simulink model "linearSingleTrack_SchrammHiller"  (R2018b)
settings: Solver=VariableStepAuto  StartTime=0.0  StopTime=20  RelTol=1e-3
settings Model: Creator=utente  LastModifiedBy=utente

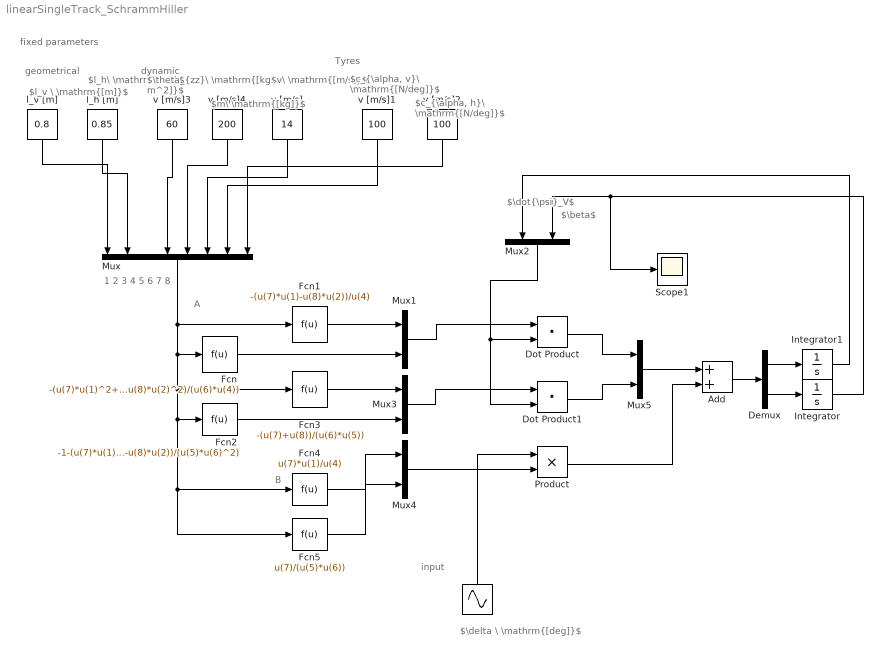
== system linearSingleTrack_SchrammHiller ==
  note: A
  note: B
  note: $\beta$
  note: $\dot{\psi}_V$
  note: 1 2 3 4 5 6 7 8
  note: dynamic
  note: geometrical
  note: Tyres
  note: $v\ \mathrm{[m/s]}$
  note: $l_h\ \mathrm{[m]}$
  note: $l_v \ \mathrm{[m]}$
  note: fixed parameters
  note: $\delta \ \mathrm{[deg]}$
  note: input
  note: $c_{\alpha, v}\ \mathrm{[N/deg]}$
  note: $c_{\alpha, h}\ \mathrm{[N/deg]}$
  note: $\theta_{zz}\ \mathrm{[kg. m^2]}$
  note: $m\ \mathrm{[kg]}$
  " " : Sin  Amplitude=10  Frequency=2*pi/5  SampleTime=0
  Add : Sum
  Demux : Demux  Outputs=2
  Dot Product : DotProduct  InputSameDT=on  OutDataTypeStr=Inherit: Inherit via internal rule
  Dot Product1 : DotProduct  InputSameDT=on  OutDataTypeStr=Inherit: Inherit via internal rule
  Fcn : Fcn  Expr=-(u(7)*u(1)^2+u(8)*u(2)^2)/(u(6)*u(4))
  Fcn1 : Fcn  Expr=-(u(7)*u(1)-u(8)*u(2))/u(4)
  Fcn2 : Fcn  Expr=-1-(u(7)*u(1)-u(8)*u(2))/(u(5)*u(6)^2)
  Fcn3 : Fcn  Expr=-(u(7)+u(8))/(u(6)*u(5))
  Fcn4 : Fcn  Expr=u(7)*u(1)/u(4)
  Fcn5 : Fcn  Expr=u(7)/(u(5)*u(6))
  Integrator : Integrator
  Integrator1 : Integrator
  Mux : Mux  Inputs=8
  Mux{1..5} (5 alike) : Mux  Inputs=2
  Product : Product
  Scope1 : Scope
  l_h [m] : Constant  Value=0.85
  l_v [m] : Constant  Value=0.8
  v [m/s] : Constant  Value=14
  v [m/s]1 : Constant  Value=100
  v [m/s]2 : Constant  Value=100
  v [m/s]3 : Constant  Value=60
  v [m/s]4 : Constant  Value=200
  wires:
  v [m/s]1/1 -> Mux/7
  v [m/s]2/1 -> Mux/8
  v [m/s]/1 -> Mux/6
  v [m/s]3/1 -> Mux/4
  v [m/s]4/1 -> Mux/5
  Mux/1 -> Fcn3/1, Fcn5/1, Fcn4/1, Fcn2/1, Fcn/1, Fcn1/1
  Fcn1/1 -> Mux1/1
  Fcn/1 -> Mux1/2
  Fcn2/1 -> Mux3/2
  Fcn3/1 -> Mux3/1
  Mux2/1 -> Dot Product1/2, Dot Product/2
  Mux1/1 -> Dot Product/1
  Mux3/1 -> Dot Product1/1
  l_v [m]/1 -> Mux/1
  l_h [m]/1 -> Mux/2
  Fcn4/1 -> Mux4/1
  Fcn5/1 -> Mux4/2
  " "/1 -> Product/1
  Mux4/1 -> Product/2
  Product/1 -> Add/2
  Dot Product/1 -> Mux5/1
  Dot Product1/1 -> Mux5/2
  Mux5/1 -> Add/1
  Add/1 -> Demux/1
  Demux/2 -> Integrator/1
  Demux/1 -> Integrator1/1
  Integrator1/1 -> Mux2/1
  Integrator/1 -> Scope1/1, Mux2/2
